simulink library "MainController"  (R2014b)
settings: Solver=ode45  StartTime=0.0  StopTime=10.0  RelTol=1e-3
libraries: simulink x2
settings Model: Creator=Sebastian  LastModifiedBy=dan

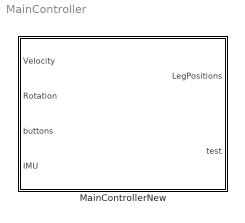
== system MainController ==
  MainControllerNew : Subsystem

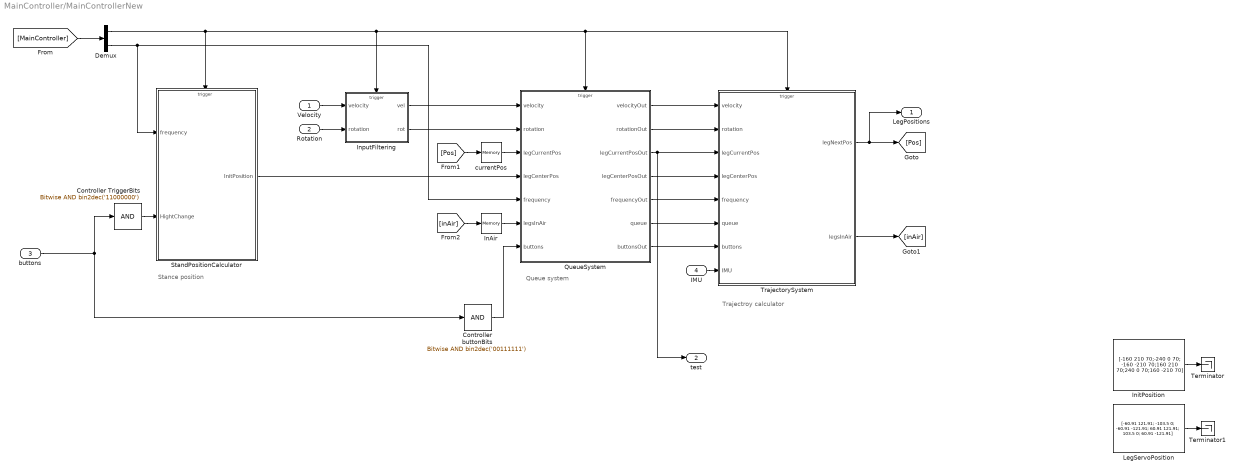
== system MainController/MainControllerNew ==
  note: Trajectroy calculator
  note: Queue system
  note: Stance position
  Velocity : Inport
  Rotation : Inport  Port=2
  buttons : Inport  Port=3
  IMU : Inport  Port=4
  Controller TriggerBits : simulink/Logic and Bit Operations/Bitwise Operator  logicop=AND  UseBitMask=on  BitMask=bin2dec('11000000')  BitMaskRealWorld=Stored Integer
  Controller buttonBits : simulink/Logic and Bit Operations/Bitwise Operator  logicop=AND  UseBitMask=on  BitMask=bin2dec('00111111')  BitMaskRealWorld=Stored Integer
  Demux : Demux  Outputs=2
  InAir : Memory  X0=zeros(6,1)  InheritSampleTime=on
  InitPosition : Constant  Value=[-160 210 70;-240 0 70; -160 -210 70;160 210 70;240 0 70;160 -210 70]
  InputFiltering : Subsystem
  LegServoPosition : Constant  Value=[-60.91 121.91; -103.5 0; -60.91 -121.91; 60.91 121.91; 103.5 0; 60.91 -121.91]
  QueueSystem : Subsystem
  StandPositionCalculator : Subsystem
  Terminator : Terminator
  Terminator1 : Terminator
  TrajectorySystem : Subsystem
  currentPos : Memory  X0=[-160 210 70;-240 0 70; -160 -210 70;160 210 70;240 0 70;160 -210 70]  InheritSampleTime=on
  LegPositions : Outport
  test : Outport  Port=2
  wires:
  [MainController] -> Demux/1
  Demux/1 -> InputFiltering/Trigger, TrajectorySystem/Trigger, QueueSystem/Trigger, StandPositionCalculator/Trigger
  buttons/1 -> Controller buttonBits/1, Controller TriggerBits/1
  Controller TriggerBits/1 -> StandPositionCalculator/2(HightChange)
  InitPosition/1 -> Terminator/1
  LegServoPosition/1 -> Terminator1/1
  [Pos] -> currentPos/1
  TrajectorySystem/1(legNextPos) -> LegPositions/1, [Pos]
  StandPositionCalculator/1(InitPosition) -> QueueSystem/4(legCenterPos)
  currentPos/1 -> QueueSystem/3(legCurrentPos)
  QueueSystem/1(velocityOut) -> TrajectorySystem/1(velocity)
  QueueSystem/5(frequencyOut) -> TrajectorySystem/5(frequency)
  QueueSystem/4(legCenterPosOut) -> TrajectorySystem/4(legCenterPos)
  QueueSystem/3(legCurrentPosOut) -> test/1, TrajectorySystem/3(legCurrentPos)
  QueueSystem/2(rotationOut) -> TrajectorySystem/2(rotation)
  QueueSystem/6(queue) -> TrajectorySystem/6(queue)
  QueueSystem/7(buttonsOut) -> TrajectorySystem/7(buttons)
  Demux/2 -> StandPositionCalculator/1(frequency), QueueSystem/5(frequency)
  InAir/1 -> QueueSystem/6(legsInAir)
  TrajectorySystem/2(legsInAir) -> [inAir]
  Controller buttonBits/1 -> QueueSystem/7(buttons)
  IMU/1 -> TrajectorySystem/8(IMU)
  [inAir] -> InAir/1
  InputFiltering/1(vel) -> QueueSystem/1(velocity)
  InputFiltering/2(rot) -> QueueSystem/2(rotation)
  Rotation/1 -> InputFiltering/2(rotation)
  Velocity/1 -> InputFiltering/1(velocity)

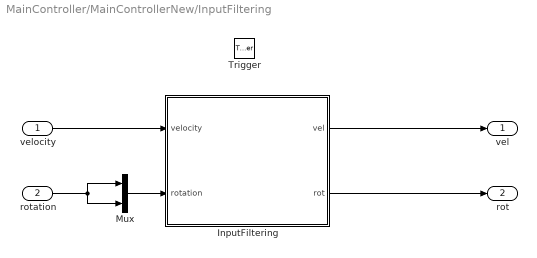
== system MainController/MainControllerNew/InputFiltering ==
  velocity : Inport
  rotation : Inport  Port=2
  Trigger : TriggerPort  PortDimensions=1
  InputFiltering : MATLAB Function  TreatAsAtomicUnit=on
  Mux : Mux  Inputs=2
  vel : Outport
  rot : Outport  Port=2
  wires:
  velocity/1 -> InputFiltering/1(velocity)
  InputFiltering/1(vel) -> vel/1
  InputFiltering/2(rot) -> rot/1
  Mux/1 -> InputFiltering/2(rotation)
  rotation/1 -> Mux/2, Mux/1

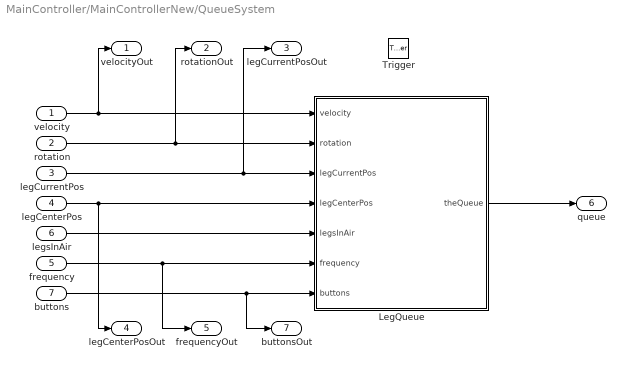
== system MainController/MainControllerNew/QueueSystem ==
  velocity : Inport
  rotation : Inport  Port=2
  legCurrentPos : Inport  Port=3
  legCenterPos : Inport  Port=4
  frequency : Inport  Port=5
  legsInAir : Inport  Port=6
  buttons : Inport  Port=7
  Trigger : TriggerPort  PortDimensions=1
  LegQueue : MATLAB Function  TreatAsAtomicUnit=on
  velocityOut : Outport
  rotationOut : Outport  Port=2
  legCurrentPosOut : Outport  Port=3
  legCenterPosOut : Outport  Port=4
  frequencyOut : Outport  Port=5
  queue : Outport  Port=6
  buttonsOut : Outport  Port=7
  wires:
  legCurrentPos/1 -> legCurrentPosOut/1, LegQueue/3(legCurrentPos)
  legCenterPos/1 -> legCenterPosOut/1, LegQueue/4(legCenterPos)
  legsInAir/1 -> LegQueue/5(legsInAir)
  LegQueue/1(theQueue) -> queue/1
  rotation/1 -> rotationOut/1, LegQueue/2(rotation)
  frequency/1 -> frequencyOut/1, LegQueue/6(frequency)
  buttons/1 -> buttonsOut/1, LegQueue/7(buttons)
  velocity/1 -> velocityOut/1, LegQueue/1(velocity)

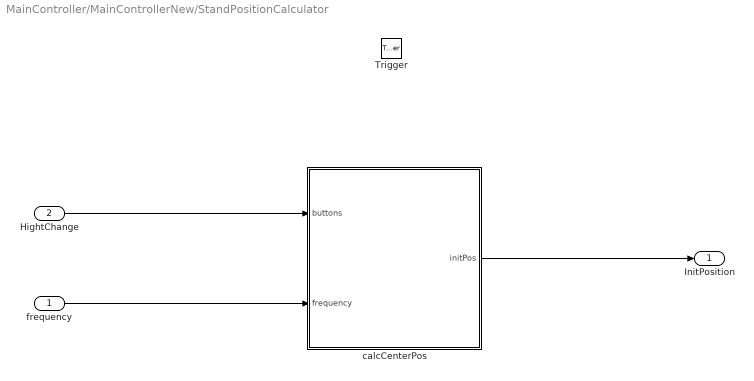
== system MainController/MainControllerNew/StandPositionCalculator ==
  frequency : Inport
  HightChange : Inport  Port=2
  Trigger : TriggerPort  PortDimensions=1
  calcCenterPos : MATLAB Function  TreatAsAtomicUnit=on
  InitPosition : Outport
  wires:
  calcCenterPos/1(initPos) -> InitPosition/1
  HightChange/1 -> calcCenterPos/1(buttons)
  frequency/1 -> calcCenterPos/2(frequency)

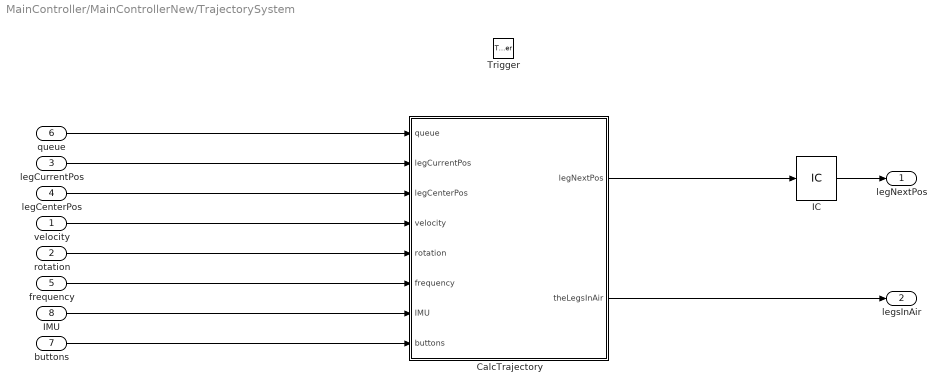
== system MainController/MainControllerNew/TrajectorySystem ==
  velocity : Inport
  rotation : Inport  Port=2
  legCurrentPos : Inport  Port=3
  legCenterPos : Inport  Port=4
  frequency : Inport  Port=5
  queue : Inport  Port=6
  buttons : Inport  Port=7
  IMU : Inport  Port=8
  Trigger : TriggerPort  PortDimensions=1
  CalcTrajectory : MATLAB Function  TreatAsAtomicUnit=on
  IC : InitialCondition  Value=[-160 210 70;-240 0 70; -160 -210 70;160 210 70;240 0 70;160 -210 70]
  legNextPos : Outport
  legsInAir : Outport  Port=2
  wires:
  legCenterPos/1 -> CalcTrajectory/3(legCenterPos)
  CalcTrajectory/2(theLegsInAir) -> legsInAir/1
  legCurrentPos/1 -> CalcTrajectory/2(legCurrentPos)
  queue/1 -> CalcTrajectory/1(queue)
  velocity/1 -> CalcTrajectory/4(velocity)
  IC/1 -> legNextPos/1
  CalcTrajectory/1(legNextPos) -> IC/1
  rotation/1 -> CalcTrajectory/5(rotation)
  frequency/1 -> CalcTrajectory/6(frequency)
  IMU/1 -> CalcTrajectory/7(IMU)
  buttons/1 -> CalcTrajectory/8(buttons)

== matlab function MainController/MainControllerNew/StandPositionCalculator/calcCenterPos ==
  data: buttons input; initPos output; frequency input
function initPos = calcCenterPos(buttons, frequency)
%This function calculates the leg center positions accoridng to the current
%chosen height. Initial height is 70 and can be increased/decreased with
%the indexfinger buttons on the controller. The center positions are saved
%in "radius" as a radius in cylindircal coordinates corresponding to a
%height*10 from their index. By knowing the sevos positions and angles the carteesian
%coordinates can be calculated.




persistent height
persistent radius
persistent servoPos
persistent servoAngle
persistent centerPos

if isempty(servoAngle)
    servoAngle = getServoAngle();
end
if isempty(servoPos)
    servoPos = getServoPos();
end
if isempty(height)
    height = 70;
end
if isempty(radius)
    radius = getLegCenter();
end
if isempty(centerPos)
    centerPos = zeros(6,3);
end

%Check if hight alteration buttons are clicked.
if buttons == 128
    heightChange = -1;
elseif buttons == 64
    heightChange = 1;
else
    heightChange = 0;
end

if heightChange ~= 0 || centerPos(1,3) == 0;
    
    %change the height according to button presses. 20mm of height per second
    %button is pressed. Also limit the height.
    height = limit(height + heightChange*10/frequency);

    %Calculate the radius appropriate for the current height. The radius is
    %linear interpolated between the hard values in "radius"
    r = interpolateR(radius, height);

    %Calculate the careesian cordinate corresponding to that radius for each servo.
    initPos =          [servoPos(1,1) + r * cosd(servoAngle(1))   servoPos(1,2) + r *sind(servoAngle(1))    height;
                        servoPos(2,1) + r * cosd(servoAngle(2))   servoPos(2,2) + r *sind(servoAngle(2))    height;
                        servoPos(3,1) + r * cosd(servoAngle(3))   servoPos(3,2) + r *sind(servoAngle(3))    height;
                        servoPos(4,1) + r * cosd(servoAngle(4))   servoPos(4,2) + r *sind(servoAngle(4))    height;
                        servoPos(5,1) + r * cosd(servoAngle(5))   servoPos(5,2) + r *sind(servoAngle(5))    height;
                        servoPos(6,1) + r * cosd(servoAngle(6))   servoPos(6,2) + r *sind(servoAngle(6))    height];
else
    initPos = centerPos;
end
end

function y = limit(height)
if height > 150
    y = 150;
elseif height < 30
    y = 30;
else
    y = height;
end

end

== matlab function MainController/MainControllerNew/InputFiltering/InputFiltering ==
  data: velocity input; vel output; rotation input; rot output
function [vel, rot] = fcn(velocity, rotation)


%The joysticks might send positions not equal to 0 when at middle position.
%Use this function to set an interval for middle position.
[vel, rot] = ControlStationary(velocity, rotation);

%In order for the robot not to move akwardly rotation is limited during
%walk.
[vel, rot] = LimitRotationDuringWalk(vel, rot);

end

== matlab function MainController/MainControllerNew/QueueSystem/LegQueue ==
  data: theQueue output; velocity input; rotation input; legCurrentPos input; legCenterPos input; legsInAir input; frequency input; buttons input
function theQueue  = LegQueue(velocity, rotation, legCurrentPos, legCenterPos, legsInAir, frequency, buttons)
%The task of this function is to create a queue of legs to move based on
%what leg is furthest from the main body. Different modes exist and mode 1
%is the working one.


persistent mode

if isempty(mode)
    mode = 1;
end

if buttons ~= 0
    mode = changeMode(mode, buttons);
end

%The joysticks might send positions not equal to 0 when at middle position.
%Use this function to set an interval for middle position.
[velocity, rotation] = ControlStationary(velocity, rotation);


if mode == 2

    velocity = velocity/10;

    rotationAngle = rotation(1)/40;
    rotationMatrix = [cosd(-rotationAngle) -sind(-rotationAngle); sind(-rotationAngle) cosd(-rotationAngle)];

    legTempPos = legCurrentPos;
    queue = zeros(2,6);

    if sum(velocity) == 0 && rotationAngle == 0
        legdiff = zeros(1,6);

        for i = 1:6
            if legsInAir(i) == 1
                legdiff(i) = -1;
            else 
                legdiff(i) = sqrt(sum((legCurrentPos(i,:) - legCenterPos(i,:)).^2));
            end
        end

        queue(2,:) = [20 20 20 20 20 20];

        for i = 1:6
            [~, pos] = max(legdiff);
            queue(1,i) = pos;
            legdiff(pos) = -2;
        end
    else

        tempQueue = zeros(2,6);

        for i = 1:6
            if legsInAir(i) == 1
                tempQueue(1,i) = 500;
            else
                while ~outsideBoundary(legTempPos(i,:), i, legCurrentPos)

                    legTempPos(i,1:2) = (legTempPos(i,1:2) - velocity(1:2,1)') * rotationMatrix;
                    tempQueue(1,i) = tempQueue(1,i) + 0.1;

                 end
            end

        end

        for i = 1:6
            [value, pos] = min(tempQueue(1,:));
            queue(:,i) = [pos, value];
            tempQueue(1,pos) = 100000;
        end
    end
elseif mode == 1
    
    %buffer
    legdiff = zeros(1,6);

    %the rotation matrix is usually used to calculate where to put legs durin
    %rotation. Though here it will be used to determine where legs are moving
    %towards.
    rotationAngle = rotation(1)/(4);
    antiRotationMatrix = [cosd(rotationAngle) -sind(rotationAngle) 0; sind(rotationAngle) cosd(rotationAngle) 0; 0 0 1];

    %calculate how far from their center position (plus direction we are moving) legs are. In order to skip
    %this step for legs movin in trajectories they are set to a diff of -1.
    for i = 1:6
        if legsInAir(i) == 1
            legdiff(i) = -1;
        else 
            legdiff(i) = sqrt(sum(((legCenterPos(i,1:3) + 3*(velocity(1:3)'))*antiRotationMatrix - legCurrentPos(i,1:3)).^2));
        end
    end

    %buffer the queue
    queue = zeros(2,6);


    %Create the queue of legs to move. legs with largest diff from previous
    %caculation are put in front.
    for i = 1:6
        [~, pos] = max(legdiff);
        queue(1,i) = pos;
        legdiff(pos) = -2;
    end
elseif mode == 3
    %buffer
    legdiff = zeros(1,6);
    
    %the rotation matrix is usually used to calculate where to put legs durin
    %rotation. Though here it will be used to determine where legs are moving
    %towards.    
    rotationAngle = rotation(1)/4;
    antiRotationMatrix = [cosd(rotationAngle) -sind(rotationAngle) 0; sind(rotationAngle) cosd(rotationAngle) 0; 0 0 1];
    rotationAngle = rotationAngle/10;
    rotationMatrix = [cosd(-rotationAngle) -sind(-rotationAngle); sind(-rotationAngle) cosd(-rotationAngle)];

    %calculate how far from their center position (plus direction we are moving) legs are. In order to skip
    %this step for legs movin in trajectories they are set to a diff of -1.
    for i = 1:6
        if legsInAir(i) == 1
            legdiff(i) = -1;
        else 
            legdiff(i) = sqrt(sum(((legCenterPos(i,1:3) + 3*(velocity(1:3)'))*antiRotationMatrix^3 - legCurrentPos(i,1:3)).^2));
        end
    end

    %buffer the queue
    queue = zeros(2,6);


    %Create the queue of legs to move. legs with largest diff from previous
    %caculation are put in front.
    for i = 1:6
        [~, pos] = max(legdiff);
        queue(1,i) = pos;
        legdiff(pos) = -2;
    end
    
    %resolution 0.1s
    velocity = velocity/10;
    legTempPos = legCurrentPos;
    
    
    %second row of the queue contains data for how many 0.1s period until
    %the leg will violate a boundary. That is calcualted here
    if sum(velocity) == 0 && rotationAngle == 0
        queue(2,:) = ones(1,6)*500;
    else    
        for i = 1:6
            if legsInAir(queue(1,i)) == 1
                queue(2,i) = 500;
            else
                while ~outsideBoundary(legTempPos(queue(1,i),:), queue(1,i), legCurrentPos)

                    legTempPos(queue(1,i),1:2) = (legTempPos(queue(1,i),1:2) - velocity(1:2,1)') * rotationMatrix;
                    queue(2,queue(1,i)) = queue(2,queue(1,i)) + 0.1;
                 end
            end
        end
    end
        
else
    queue = [1 2 3 4 5 6;20 20 20 20 20 20];
end
theQueue = queue;

== matlab function MainController/MainControllerNew/TrajectorySystem/CalcTrajectory ==
  data: legNextPos output; queue input; legCurrentPos input; legCenterPos input; theLegsInAir output; velocity input; rotation input; frequency input; IMU input; buttons input
function [legNextPos, theLegsInAir] = calcTrajectories(queue, legCurrentPos, legCenterPos, velocity, rotation, frequency, IMU, buttons)
%This is the function that determines next positions for each leg. This can
%be done in several different modes. mode 1 and 6 are the currently working
%ones.

persistent legsInAir;
persistent trajectory;
persistent counter;
persistent height;
persistent heightCounter;
persistent boundary;
persistent floorAngle;
persistent mode;

IMU = IMU(1:2)';

%Initiation of persistent variables
if isempty(legsInAir)
    legsInAir = zeros(6,1);
end
if isempty(trajectory)
    trajectory = zeros(3,50,6);
end
if isempty(counter)
    counter = ones(6,1);
end
if isempty(height)
    height = legCenterPos(1,3);
end
if isempty(heightCounter)
    heightCounter = 0;
end
if isempty(boundary)
    boundary = getBoundary();
end
if isempty(floorAngle)
    floorAngle = [0 0];
end
if isempty(mode)
    mode = 1;
end


if buttons ~= 0
    mode = changeMode(mode, buttons);
end

%Detemine if there has been a difference in height since last sample. The
%counter is used to determine if the button for hight alteration has been
%purposly realeased since it is a bit inconsistent.
heightDiff = legCenterPos(1,3) - height;
if heightDiff == 0
    heightCounter = heightCounter + 1;
else
    heightCounter = 0;
end

%update the current height
height = legCenterPos(1,3);

%alter trajectories for height differences between samples.
trajectory(3,:,:) = trajectory(3,:,:) + heightDiff;

legNextPos = legCurrentPos;

if mode <= 3


    %No moving velocity or rotation, nor height movement for six samples will
    %result in moving legs back to center position for that height.
    if sqrt(sum(velocity.^2)) == 0 && abs(rotation(1)) == 0 && heightCounter > 6;

        %During standing still only make trajectorys one leg at a
        %time.
        if sum(legsInAir) < 1

            %Go through the queue to determine if legs need to be moved to
            %center position.
            for i=1:6
                legID = queue(1,i);

                %If leg is not already in air (made for the ability to move
                %several legs during standstill).
                if legsInAir(queue(1,i)) == 0
                    %determine if legs are far away from center position.
                    if ~isEqualPos(legCurrentPos(legID,:), legCenterPos(legID,:))

                        %If leg is allowed to be lifted (made for the ability to move
                        %several legs during standstill).
                        if liftable(legsInAir, legID)

                            %Create a trajectory in order to move leg back to
                            %center position.
                            trajectory(:,:,legID) = makeLiftTrajectory(legCurrentPos(legID,:), legCenterPos(legID,:), frequency, 500);
                            legsInAir(legID) = 1;
                            break;

                        end
                    end
                end
            end
        end

    %movement by either velocity or rotation. Will result in a walking
    %hexapod
    elseif sqrt(sum(velocity.^2)) > 0 || abs(rotation(1)) > 0

        %Determine how many legs the hexapod is allowed to move simultaniously
        %based on the velocity and rotation.
        queue
        legsInAir
        [movableLegs, velocity, rotation, nerf, time] = legLimit(velocity, rotation, queue, legsInAir, mode);

        %matrices used for tha rotation of leg positions. In order not to
        %rotate to ferocious there is a division. rotationdegrees per second is
        %rotationvalue divided by 4
        rotationAngle = (0.5 + 0.5*(3-movableLegs)^2)*rotation(1)/4;
        antiRotationMatrix = [cosd(rotationAngle) -sind(rotationAngle) 0; sind(rotationAngle) cosd(rotationAngle) 0; 0 0 1];
        rotationAngle = rotation(1)/(4*frequency);
        rotationMatrix = [cosd(-rotationAngle) -sind(-rotationAngle) 0; sind(-rotationAngle) cosd(-rotationAngle) 0; 0 0 1];


        if mode == 2

            %If there is ability to lift additional legs it is done here.
            if sum(legsInAir) < movableLegs

                %Only check if the 2 first in the queue can be lifted. This is to
                %not forget legs behind because of unliftablility.
                for i = 1:6
                    legID = queue(1,i);
                    if liftable(legsInAir, legID) && legsInAir(legID) == 0
                        goalPos = calcGoalPos(legCenterPos, legID, velocity, rotation(1), legCurrentPos, movableLegs);
                        if ~isequal(legCurrentPos(legID,:), goalPos)
                            trajectory(:,:,legID) = makeLiftTrajectory(legCurrentPos(legID,:), goalPos, frequency, time);
                            legsInAir(legID) = 1;
                        end
                        if sum(legsInAir) >= movableLegs
                            break;
                        end
                    end
                end
            end
        elseif mode == 3

        %If there is ability to lift additional legs it is done here.
        if sum(legsInAir) < movableLegs

            %Only check if the 2 first in the queue can be lifted. This is to
            %not forget legs behind because of unliftablility.
            for i = 1:2
                legID = queue(1,i);
                if liftable(legsInAir, legID) && legsInAir(legID) == 0
                    goalPos = calcGoalPos(legCenterPos, legID, velocity, rotation(1), legCurrentPos, movableLegs);
                    if ~isequal(legCurrentPos(legID,:), goalPos)
                        trajectory(:,:,legID) = makeLiftTrajectory(legCurrentPos(legID,:), goalPos, frequency, 750);
                        legsInAir(legID) = 1;
                    end
                    if sum(legsInAir) >= movableLegs
                        break;
                    end
                end
            end
        end
        elseif mode == 1
            
            %If there is ability to lift additional legs it is done here.
            if sum(legsInAir) < movableLegs

                %Only check if the 2 first in the queue can be lifted. This is to
                %not forget legs behind because of unliftablility.
                for i = 1:2
                    legID = queue(1,i);
                    if liftable(legsInAir, legID) && legsInAir(legID) == 0
                        if ~isequal(legCurrentPos(legID,:), (legCenterPos(legID,:) + (0.5 + 0.5*(3-movableLegs)^2)*(velocity'))*antiRotationMatrix)
                            trajectory(:,:,legID) = makeLiftTrajectory(legCurrentPos(legID,:), (legCenterPos(legID,:) + (0.5 + 0.5*(3-movableLegs)^2)*(velocity'))*antiRotationMatrix, frequency, 650);
                            legsInAir(legID) = 1;
                            break;
                        end
                    end
                end
            end
        end
            

        %Also move the legs not lifted in opposite direction of movement in
        %order to create movement.
        for i = 1:6
            if legsInAir(i) == 0 && nerf == 0;
                legNextPos(i,:) = (legCurrentPos(i,:) - (velocity/(frequency))')*rotationMatrix + [0 0 heightDiff];
            end
        end

    % only height movement. (needs a fix for moving legs when getting to far
    % from center position)
    else
        for i = 1:6
            if legsInAir(i) == 0
                legNextPos(i,:) = legCurrentPos(i,:) + [0 0 heightDiff];
            end
        end
    end


    %carry out trajectory movement for lifted legs
    if sum(legsInAir) ~= 0
        for i = 1:6
            if legsInAir(i) == 1
                legNextPos(i,:) = trajectory(:,counter(i),i);
                counter(i) = counter(i) + 1;

                %Determine if leg is on ground. In that case terminate
                %trajectroy movement.
                if groundTouch(legNextPos(i,:), legCenterPos(i,:))
                    legsInAir(i) = 0;
                    counter(i) = 1;
                end
            end
        end
    end
end

%This part uses mode 5 & 6. This is for balancing. The IMU data is divided
%by 5 to get a gain of 0.2 to get a stable P controller.
if mode >= 5 && sum(abs(IMU)) >= 1
    legNextPos = floorCompensate(legNextPos, IMU/5, mode);
    floorAngle = floorAngle + IMU(1,1:2)/5;
end


%Problems with positions as NaN has occured. in order for the full
%controller not to collapse this just rewing the NaN value back to previous
%value.
for i=1:6
    for j= 1:3
        if isnan(legNextPos(i,j))
            legNextPos(i,j) = legCurrentPos(i,j);
        end
    end
end

%tell system whitch legs are in the air.
theLegsInAir = legsInAir;

end
